simulink model "sample_model"  (R2023a)
settings: Solver=FixedStepAuto  StartTime=0.0  StopTime=10.0  RelTol=1e-3
libraries: androiduilib x9, androidsensorlib x3, androidaudiovideolib x2, androidcommunicationlib x2
settings Model: Creator=ragha  LastModifiedBy=Shesh
settings OptimizationCC: EnhancedBackFolding=on  PassReuseOutputArgsAs=Individual arguments  ZeroExternalMemoryAtStartup=off  ZeroInternalMemoryAtStartup=off  MaxStackSize=64  OptimizeBlockOrder=speed  DifferentSizesBufferReuse=on  OptimizationCustomize=off  EfficientTunableParamExpr=on
settings DebuggingCC: ParameterTunabilityLossMsg=error
settings HardwareCC: ProdBitPerPointer=32  ProdBitPerSizeT=32  ProdBitPerPtrDiffT=32  ProdLargestAtomicInteger=Long  ProdLargestAtomicFloat=Double  ProdWordSize=32  ProdHWDeviceType=ARM Compatible->ARM Cortex
settings SFSimCC: MATLABDynamicMemAlloc=off
settings RTWCC: Description=Embedded Coder  SystemTargetFile=ert.tlc  HardwareBoard=Android Device  TLCOptions="-aInlineSetEventsForThisBaseRateFcn=TLC_FALSE -aSuppressMultiTaskScheduler=TLC_FALSE  -aRateBasedStepFcn=0"  TemplateMakefile=ert_default_tmf  RTWVerbose=off  Toolchain=Android SDK/NDK Tools
settings CodeAppCC: ForceParamTrailComments=on  IgnoreCustomStorageClasses=off  OperatorAnnotations=on  SimulinkDataObjDesc=on  SFDataObjDesc=on  InsertBlockDesc=on

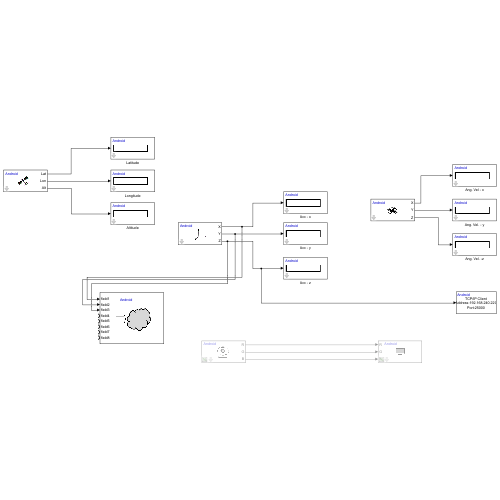
[thumbnail: Simulink's stored preview of the top-level diagram]
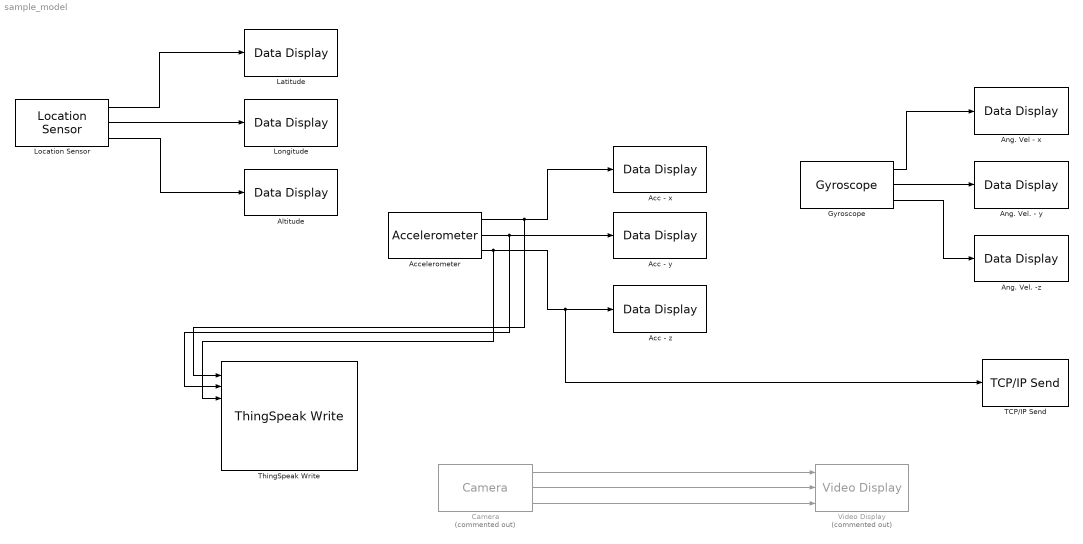
== system sample_model ==
  Acc - x : androiduilib/Data Display  DataDisplayId=sample_model/Acc_-_x  Format=Float  Precision=6  SimulateUsing=Code generation  blockPlatform=Android
  Acc - y : androiduilib/Data Display  DataDisplayId=sample_model/Acc_-_y  Format=Float  Precision=6  SimulateUsing=Code generation  blockPlatform=Android
  Acc - z : androiduilib/Data Display  DataDisplayId=sample_model/Acc_-_z  Format=Float  Precision=6  SimulateUsing=Code generation  blockPlatform=Android
  Accelerometer : androidsensorlib/Accelerometer  OutputVector=off  SampleTime=1  BlockPlatform=Android
  Altitude : androiduilib/Data Display  DataDisplayId=sample_model/Altitude  Format=Float  Precision=6  SimulateUsing=Code generation  blockPlatform=Android
  Ang. Vel - x : androiduilib/Data Display  DataDisplayId=sample_model/Ang._Vel_-_x  Format=Float  Precision=6  SimulateUsing=Code generation  blockPlatform=Android
  Ang. Vel. - y : androiduilib/Data Display  DataDisplayId=sample_model/Ang._Vel._-_y  Format=Float  Precision=6  SimulateUsing=Code generation  blockPlatform=Android
  Ang. Vel. -z : androiduilib/Data Display  DataDisplayId=sample_model/Ang._Vel._-z  Format=Float  Precision=6  SimulateUsing=Code generation  blockPlatform=Android
  Camera : androidaudiovideolib/Camera  Commented=on  CameraLocation=Back  CameraResolutions=Back - 640x480  Width=640  Height=480  SampleTime=0.001  BlockPlatform=Android
  Gyroscope : androidsensorlib/Gyroscope  OutputVector=off  SampleTime=0.1  BlockPlatform=Android
  Latitude : androiduilib/Data Display  DataDisplayId=sample_model/Latitude  Format=Float  Precision=6  SimulateUsing=Code generation  blockPlatform=Android
  Location Sensor : androidsensorlib/Location Sensor  OutputVector=off  SampleTime=0.1  BlockPlatform=Android
  Longitude : androiduilib/Data Display  DataDisplayId=sample_model/Longitude  Format=Float  Precision=6  SimulateUsing=Code generation  blockPlatform=Android
  TCP/IP Send : androidcommunicationlib/TCP//IP Send  TCPSendId=sample_model/TCP//IP_Send  Mode_=Client  LocalServerPort_=25000  RemoteAddr_=192.168.240.220  RemoteServerPort_=25000  ClientPortBindingSelection_=off  ClientPortToBind_=35000  BlockingMode_=off  BlockTimeout_=0.1
  ThingSpeak Write : androidcommunicationlib/ThingSpeak Write  ChannelID=2272726  WriteAPIKey=F3AJHHWU1CZNX648  NumberOfFields=8  UpdateInterval=30  LocationEnabled=off  LocationSource=Block dialog  BlockPlatform=Android
  Video Display : androidaudiovideolib/Video Display  Commented=on  BlockPlatform=Android
  wires:
  Camera/1 -> Video Display/1
  Camera/2 -> Video Display/2
  Accelerometer/1 -> ThingSpeak Write/1, Acc - x/1
  Accelerometer/2 -> ThingSpeak Write/2, Acc - y/1
  Accelerometer/3 -> ThingSpeak Write/3, TCP/IP Send/1, Acc - z/1
  Location Sensor/2 -> Longitude/1
  Location Sensor/1 -> Latitude/1
  Location Sensor/3 -> Altitude/1
  Gyroscope/1 -> Ang. Vel - x/1
  Gyroscope/2 -> Ang. Vel. - y/1
  Gyroscope/3 -> Ang. Vel. -z/1
  Camera/3 -> Video Display/3
